simulink model "teleop2_arrows_32"  (Simulink 10.3)
settings: Solver=ode1  StartTime=0.0  StopTime=inf  FixedStep=0.01  RelTol=1e-3  EnableMultiTasking=on
undefined symbols (not defined in the file): gcbh, HIL, Host, JPEG, qc_get_step_size, Video3D, video_display_show
libraries: quarc_library x18
settings Model: Creator=drmadill  LastModifiedBy=Rohan  SimulationMode=external  ExtModeTrigDuration=2
settings SolverCC: PositivePriorityOrder=on
settings DataIOCC: LimitDataPoints=on
settings OptimizationCC: LifeSpan=auto
settings DebuggingCC: SolverPrmCheckMsg=warning
settings HardwareCC: ProdLargestAtomicInteger=Long  ProdLargestAtomicFloat=Double  ProdIntDivRoundTo=Zero  ProdEndianess=LittleEndian  ProdHWDeviceType=ARM Compatible->ARM Cortex
settings RTWCC: Description=QUARC Linux Raspberry Pi 3 Target (QBot 2e) Using Toolchain  SystemTargetFile=quarc_linux_pi_3.tlc  TemplateMakefile=quarc_default_tmf  Toolchain=QUARC linux_pi_3 | gmake (64-bit Windows)  BuildConfiguration=Faster Runs
settings STFCustomTargetCC: ConcurrentExecutionCompliant=on  UseToolchainInfoCompliant=on  SystemTargetFile=quarc_linux_pi_3.tlc
settings GRTTargetCC: ParMdlRefBuildCompliant=off  CompOptLevelCompliant=off  MatFileLogging=off  CPPClassGenCompliant=off  ExtMode=on  ExtModeMexFile=quarc_comm  ExtModeMexArgs='-w -d /tmp -uri %u', 'tcpip://192.168.2.32:17001'
settings ConfigComp: CovSFcnEnable=off

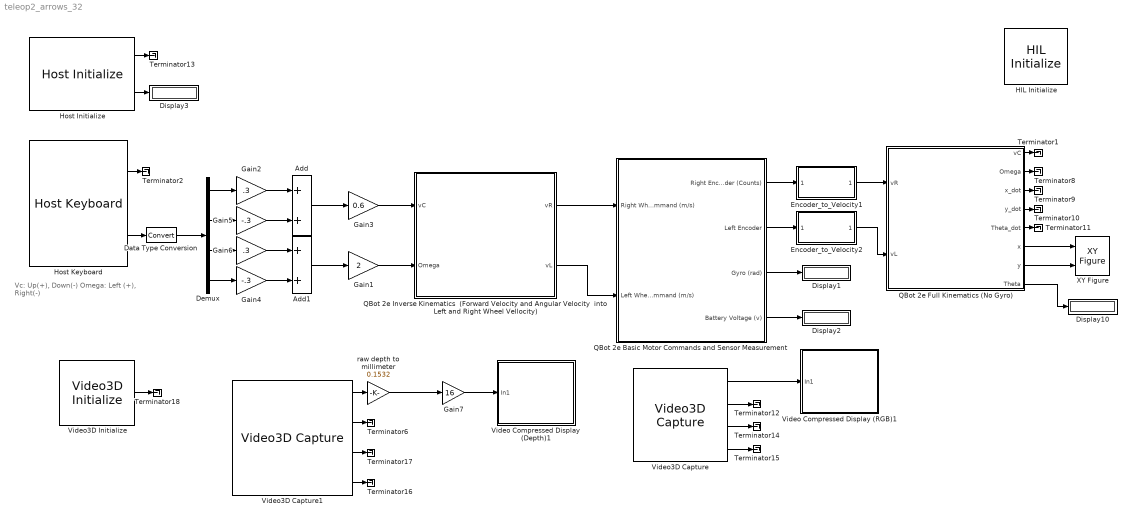
== system teleop2_arrows_32 ==
  note: Vc: Up(+), Down(-)
      | Omega: Left (+), Right(-)
  Add : Sum
  Add1 : Sum
  Data Type Conversion : DataTypeConversion
  Demux : Demux
  Display{1..3,10} (4 alike) : Display
  Encoder_to_Velocity1 : Subsystem
  Encoder_to_Velocity2 : Subsystem
  Gain1 : Gain  Gain=2
  Gain2 : Gain  Gain=.3
  Gain3 : Gain  Gain=0.6
  Gain4 : Gain  Gain=-.3
  Gain5 : Gain  Gain=-.3
  Gain6 : Gain  Gain=.3
  Gain7 : Gain  Gain=16  OutDataTypeStr=uint16
  HIL Initialize : quarc_library/Data Acquisition/Generic/Configuration/HIL Initialize  Priority=-99  object_name=HIL-1  board_type=qbot2e  board_number=0  board_options=pwm0_en=1;pwm0_pin=12;pwm1_en=1;pwm1_pin=13;  exclusive=off  active=off  hardware_clocks=[]  clock_modes=[]  initial_clock_frequencies=[]  set_clock_params_at_start=off  set_clock_params_at_switch_in=off  set_clock_frequencies_at_start=off  set_clock_frequencies_at_switch_in=off  analog_input_channels=[0:5]  analog_input_configurations=[]  analog_input_maximums=[16.5 3.3 3.3 3.3 3.3 3.3]  analog_input_minimums=[0 0 0 0 0 0]  set_analog_input_params_at_start=off  set_analog_input_params_at_switch_in=off  analog_output_channels=[]  analog_output_maximums=[]  analog_output_minimums=[]  initial_analog_outputs=[]  final_analog_outputs=[]  watchdog_analog_outputs=[]  set_analog_output_params_at_start=off  set_analog_output_params_at_switch_in=off  set_analog_outputs_at_start=off  set_analog_outputs_at_switch_in=off  set_analog_outputs_at_terminate=off  set_analog_outputs_at_switch_out=off  set_analog_outputs_on_watchdog=off  digital_input_channels=[28:58]  digital_output_channels=[28:31]  digital_output_configuration=[]  initial_digital_outputs=[0]  final_digital_outputs=[0]  watchdog_digital_outputs=[]  set_digital_output_params_at_start=off  set_digital_output_params_at_switch_in=off  set_digital_outputs_at_start=on  set_digital_outputs_at_switch_in=off  set_digital_outputs_at_terminate=on  set_digital_outputs_at_switch_out=off  set_digital_outputs_on_watchdog=off  encoder_channels=[0:1]  quadrature=[4]  encoder_filter_frequency=[]  initial_encoder_counts=[0]  set_encoder_params_at_start=on  set_encoder_params_at_switch_in=off  set_encoder_counts_at_start=on  set_encoder_counts_at_switch_in=off  pwm_channels=[0:1]  pwm_modes=0  pwm_frequency=100e6 / 4095  pwm_configuration=[0]  pwm_alignment=[0]  pwm_polarity=[1]  pwm_leading_deadband=[]  pwm_trailing_deadband=[]  initial_pwm_outputs=[0]  final_pwm_outputs=[0]  watchdog_pwm_outputs=[]  set_pwm_params_at_start=on  set_pwm_params_at_switch_in=off  set_pwm_outputs_at_start=on  set_pwm_outputs_at_switch_in=off  set_pwm_outputs_at_terminate=on  set_pwm_outputs_at_switch_out=off  set_pwm_outputs_on_watchdog=off  other_output_channels=[2000:2001 14000 16000]  initial_other_outputs=[0 0 0 7]  final_other_outputs=[0 0 0 7]  watchdog_other_outputs=[]  set_other_outputs_at_start=on  set_other_outputs_at_switch_in=off  set_other_outputs_at_terminate=on  set_other_outputs_at_switch_out=off  set_other_outputs_on_watchdog=off
  Host Initialize : quarc_library/Devices/Peripherals/Host/Host Initialize  object_name=Host-1  uri_source=Use external mode communications  uri=tcpip://192.168.2.104:17001  apply_uri_to_all_configs=on  send_buffer_size=1000  receive_buffer_size=1000  thread_priority=0  run_client=on  use_window=off  window_position=[]  sample_time=qc_get_step_size  active=on
      settings: SourceProductName=QUARC Targets
  Host Keyboard : quarc_library/Devices/Peripherals/Host/Host Keyboard  object_name=Host-1  virtual_key="[38  40  37  39]"  sample_time=qc_get_step_size  enabled=on  debug_mode=off
      settings: SourceProductName=QUARC Targets
  QBot 2e Basic Motor Commands and Sensor Measurement : Subsystem
  QBot 2e Full Kinematics (No Gyro) : Subsystem
  QBot 2e Inverse Kinematics  (Forward Velocity and Angular Velocity  into Left and Right Wheel Vellocity) : Subsystem
  Terminator{1..2,6,8..18} (14 alike) : Terminator
  Video Compressed Display (Depth)1 : Subsystem  LoadFcn=set_param(gcbh, 'UserData', gcb);  StartFcn=video_display_show([gcb, '/Video Display'], 'add', gcb);  mask(Video Compressed Display){algorithm=JPEG, quality=50, sample_time=-1, use_hardware=on}
      mask prompts: algorithm "Compression algorithm:"; quality "Compression quality (0-100):"; sample_time "Sample time (seconds):"; use_hardware "Use hardware acceleration for video display"
      mask help: Displays a video stream on the host, using compression to minimize bandwidth.
      mask init:
      | qc_set_display('Video\nCompressed\nDisplay');
      settings: UndoDeleteFcn=set_param(gcbh, 'UserData', gcb);  OpenFcn=video_display_show([gcb, '/Video Display'], 'show', gcb);  PreDeleteFcn=video_display_show([gcb, '/Video Display'], 'delete');
      settings: CopyFcn=|
      | set_param(gcbh, 'UserData', gcb);
      | set_param(gcbh, 'LinkStatus', 'none');
      settings: NameChangeFcn=|
      | video_display_show([get_param(gcbh, 'UserData'), '/Video Display'], 'rename', [gcb, '/Video Display']);
      | video_display_show([gcb, '/Video Display'], 'add', gcb);
      | set_param(gcbh, 'UserData', gcb);
      mask Help: web(qc_get_block_help_path(gcb));
      mask TypeOptions algorithm: Image Compress/algorithm
      mask TypeOptions quality: Image Compress/quality
      mask TypeOptions sample_time: Video Display/sample_time
      mask TypeOptions use_hardware: Video Display/use_hardware
      mask Display:
      | patch([0.98591 0.98591 0.62618 0.59072 0.56147   0.536   0.536  0.5441 0.56912 0.59207 0.60881 0.62276 0.63527 0.64364  0.6485  0.6485 0.64706 0.64499 0.63662 0.62411 0.61232 0.59837 0.58307 0.56147   0.536   0.536  0.5441  0.5747 0.60953 0.63662 0.67001  0.7034 0.72851 0.75425 0.77927 0.80294 0.82454 0.84119 0.85865 0.87395 0.88574 0.89339  0.8969 0.89969 0.89969 0.89267  0.8816 0.87044 0.85649  0.8384 0.81824 0.80294 0.78764 0.77513 0.76676 0.75776 0.76397 0.77513 0.79178 0.80987 0.82796 0.84326 0.86207 0.98528],[0.18689 0.05522 0.05522 0.05171 0.05171    0.05 0.18338 0.18338 0.19148 0.20435 0.22298 0.24863 0.28589 0.33125 0.38138 0.55139 0.59801 0.63761 0.68189 0.72149 0.74939 0.76694 0.77855 0.79367 0.79952 0.92768 0.92768 0.92768 0.92417 0.92066 0.91364  0.9032 0.89384 0.88106 0.86594 0.85073 0.82634 0.80537 0.77855 0.74363 0.70403 0.65858 0.61079 0.59099 0.41513 0.37202 0.31847 0.29048 0.25556 0.23342  0.2102 0.19382 0.18221 0.17285 0.16943 0.16124  0.1589 0.16241 0.16709 0.17168  0.1787 0.18221 0.18689 0.18689],[0.9,0.90,0.91])
      | patch([0.536 0.52601 0.46823 0.44528 0.41603 0.39101 0.35555 0.33116 0.31451 0.29291  0.2804 0.26717 0.25322 0.23999 0.22406 0.20732 0.19337 0.17528 0.15935 0.14396 0.13217 0.11759 0.10922 0.10085 0.09671 0.09392 0.09041 0.08906 0.08906 0.09464  0.0995 0.10778 0.11894 0.13145 0.14675 0.16349 0.17672 0.19409 0.20732 0.22406 0.23999 0.26159 0.27833 0.29849 0.31793 0.33602 0.35411 0.37085 0.39245 0.41603   0.536   0.536 0.53159 0.46409   0.446 0.42026 0.39587 0.37571 0.36113 0.34925 0.34088 0.33809 0.33809 0.34088 0.34583 0.35627 0.36392 0.38129 0.39587 0.41117 0.42719 0.44672  0.4676 0.48353 0.48353 0.52394   0.536],[0.05 0.04829 0.04712 0.04712 0.04829 0.05063 0.05405 0.05873 0.06107 0.06692 0.07043 0.07619 0.08087 0.08672 0.09482 0.10652 0.11696 0.13325  0.1508 0.17168 0.19499 0.22415 0.25439 0.28472 0.31379 0.35456 0.38489 0.41513 0.58055 0.63878 0.68774 0.72149 0.75641 0.78089 0.80537 0.82859 0.84029 0.85658 0.86594 0.87404  0.8834 0.89267 0.90086 0.90788 0.91247 0.91832 0.92066   0.923 0.92651 0.92768 0.92768 0.79952 0.79952 0.79952 0.79718 0.78899 0.77153 0.75056 0.72149 0.68072 0.62249  0.5549 0.41396 0.37085 0.33242 0.28121 0.25205 0.22181 0.20552 0.19499 0.18572 0.18221 0.17753 0.17636 0.17753  0.1787  0.1787],[0.9,0.90,0.91])
      | disp('Video\nCompressed\nDisplay');
  Video Compressed Display (RGB)1 : Subsystem  LoadFcn=set_param(gcbh, 'UserData', gcb);  StartFcn=video_display_show([gcb, '/Video Display'], 'add', gcb);  mask(Video Compressed Display){algorithm=JPEG, quality=50, sample_time=-1, use_hardware=on}
      mask prompts: algorithm "Compression algorithm:"; quality "Compression quality (0-100):"; sample_time "Sample time (seconds):"; use_hardware "Use hardware acceleration for video display"
      mask help: Displays a video stream on the host, using compression to minimize bandwidth.
      mask init:
      | qc_set_display('Video\nCompressed\nDisplay');
      settings: UndoDeleteFcn=set_param(gcbh, 'UserData', gcb);  OpenFcn=video_display_show([gcb, '/Video Display'], 'show', gcb);  PreDeleteFcn=video_display_show([gcb, '/Video Display'], 'delete');
      settings: CopyFcn=|
      | set_param(gcbh, 'UserData', gcb);
      | set_param(gcbh, 'LinkStatus', 'none');
      settings: NameChangeFcn=|
      | video_display_show([get_param(gcbh, 'UserData'), '/Video Display'], 'rename', [gcb, '/Video Display']);
      | video_display_show([gcb, '/Video Display'], 'add', gcb);
      | set_param(gcbh, 'UserData', gcb);
      mask Help: web(qc_get_block_help_path(gcb));
      mask TypeOptions algorithm: Image Compress/algorithm
      mask TypeOptions quality: Image Compress/quality
      mask TypeOptions sample_time: Video Display/sample_time
      mask TypeOptions use_hardware: Video Display/use_hardware
      mask Display:
      | patch([0.98591 0.98591 0.62618 0.59072 0.56147   0.536   0.536  0.5441 0.56912 0.59207 0.60881 0.62276 0.63527 0.64364  0.6485  0.6485 0.64706 0.64499 0.63662 0.62411 0.61232 0.59837 0.58307 0.56147   0.536   0.536  0.5441  0.5747 0.60953 0.63662 0.67001  0.7034 0.72851 0.75425 0.77927 0.80294 0.82454 0.84119 0.85865 0.87395 0.88574 0.89339  0.8969 0.89969 0.89969 0.89267  0.8816 0.87044 0.85649  0.8384 0.81824 0.80294 0.78764 0.77513 0.76676 0.75776 0.76397 0.77513 0.79178 0.80987 0.82796 0.84326 0.86207 0.98528],[0.18689 0.05522 0.05522 0.05171 0.05171    0.05 0.18338 0.18338 0.19148 0.20435 0.22298 0.24863 0.28589 0.33125 0.38138 0.55139 0.59801 0.63761 0.68189 0.72149 0.74939 0.76694 0.77855 0.79367 0.79952 0.92768 0.92768 0.92768 0.92417 0.92066 0.91364  0.9032 0.89384 0.88106 0.86594 0.85073 0.82634 0.80537 0.77855 0.74363 0.70403 0.65858 0.61079 0.59099 0.41513 0.37202 0.31847 0.29048 0.25556 0.23342  0.2102 0.19382 0.18221 0.17285 0.16943 0.16124  0.1589 0.16241 0.16709 0.17168  0.1787 0.18221 0.18689 0.18689],[0.9,0.90,0.91])
      | patch([0.536 0.52601 0.46823 0.44528 0.41603 0.39101 0.35555 0.33116 0.31451 0.29291  0.2804 0.26717 0.25322 0.23999 0.22406 0.20732 0.19337 0.17528 0.15935 0.14396 0.13217 0.11759 0.10922 0.10085 0.09671 0.09392 0.09041 0.08906 0.08906 0.09464  0.0995 0.10778 0.11894 0.13145 0.14675 0.16349 0.17672 0.19409 0.20732 0.22406 0.23999 0.26159 0.27833 0.29849 0.31793 0.33602 0.35411 0.37085 0.39245 0.41603   0.536   0.536 0.53159 0.46409   0.446 0.42026 0.39587 0.37571 0.36113 0.34925 0.34088 0.33809 0.33809 0.34088 0.34583 0.35627 0.36392 0.38129 0.39587 0.41117 0.42719 0.44672  0.4676 0.48353 0.48353 0.52394   0.536],[0.05 0.04829 0.04712 0.04712 0.04829 0.05063 0.05405 0.05873 0.06107 0.06692 0.07043 0.07619 0.08087 0.08672 0.09482 0.10652 0.11696 0.13325  0.1508 0.17168 0.19499 0.22415 0.25439 0.28472 0.31379 0.35456 0.38489 0.41513 0.58055 0.63878 0.68774 0.72149 0.75641 0.78089 0.80537 0.82859 0.84029 0.85658 0.86594 0.87404  0.8834 0.89267 0.90086 0.90788 0.91247 0.91832 0.92066   0.923 0.92651 0.92768 0.92768 0.79952 0.79952 0.79952 0.79718 0.78899 0.77153 0.75056 0.72149 0.68072 0.62249  0.5549 0.41396 0.37085 0.33242 0.28121 0.25205 0.22181 0.20552 0.19499 0.18572 0.18221 0.17753 0.17636 0.17753  0.1787  0.1787],[0.9,0.90,0.91])
      | disp('Video\nCompressed\nDisplay');
  Video3D Capture : quarc_library/Multimedia/Video3D Capture  object_name=Video3D-1  stream_type=RGB  stream_index=0  resolution=640 x 480  width=640  height=480  output_format=MATLAB RGB (HxWx3)  data_type=uint8  sample_time=qc_get_step_size * ceil(0.033 / qc_get_step_size)  brightness_override=off  brightness=50.0  contrast_override=off  contrast=50.0  hue_override=off  hue=50.0  saturation_override=off  saturation=50.0  sharpness_override=off  sharpness=50.0  gamma_override=off  gamma=50.0  gain_override=off  gain=50.0  backlightcompensation_override=off  backlightcompensation=50.0  whitebalance_override=Automatic white balance  whitebalance=50.0  exposure_override=Automatic exposure  exposure=30.0  emitter=Enable laser emitter  preset=Do not set camera presets
  Video3D Capture1 : quarc_library/Multimedia/Video3D Capture  object_name=Video3D-1  stream_type=Depth  stream_index=0  resolution=640 x 480  width=640  height=480  output_format=MATLAB greyscale (HxW)  data_type=uint16  sample_time=qc_get_step_size * ceil(0.033 / qc_get_step_size)  brightness_override=off  brightness=50.0  contrast_override=off  contrast=50.0  hue_override=off  hue=50.0  saturation_override=off  saturation=50.0  sharpness_override=off  sharpness=50.0  gamma_override=off  gamma=50.0  gain_override=off  gain=50.0  backlightcompensation_override=off  backlightcompensation=50.0  whitebalance_override=Automatic white balance  whitebalance=50.0  exposure_override=Automatic exposure  exposure=30.0  emitter=Enable laser emitter  preset=Do not set camera presets
  Video3D Initialize : quarc_library/Multimedia/Video3D Initialize  object_name=Video3D-1  source=Device  identifier=0  file=sample.bag  sample_time=qc_get_step_size * ceil(0.033 / qc_get_step_size)  active=on
  XY Figure : quarc_library/Sinks/Figures/XY Figure  figure_mode=Use figure window  figure_tag=figure1  axes_tag=axes1  plot_mode=Time-based  minimum_x=-1  maximum_x=1  minimum_y=-1  maximum_y=1  buffer_size=1000  update_rate=100  initial_position="581  184  710  615"  initial_visibility=off  sample_time=-1
      settings: SourceProductName=QUARC Targets
  raw depth to millimeter : Gain  Gain=0.1532
  wires:
  Host Initialize/2 -> Display3/1
  Host Initialize/1 -> Terminator13/1
  QBot 2e Basic Motor Commands and Sensor Measurement/2(Left Encoder) -> Encoder_to_Velocity2/1(Encoder)
  QBot 2e Full Kinematics (No Gyro)/8(Theta) -> Display10/1
  QBot 2e Full Kinematics (No Gyro)/7(y) -> XY Figure/2
  QBot 2e Full Kinematics (No Gyro)/6(x) -> XY Figure/1
  Encoder_to_Velocity1/1(Velocity) -> QBot 2e Full Kinematics (No Gyro)/1(vR)
  Encoder_to_Velocity2/1(Velocity) -> QBot 2e Full Kinematics (No Gyro)/2(vL)
  QBot 2e Inverse Kinematics  (Forward Velocity and Angular Velocity  into Left and Right Wheel Vellocity)/1(vR) -> QBot 2e Basic Motor Commands and Sensor Measurement/1(Right Wheel Command (m/s))
  Gain3/1 -> QBot 2e Inverse Kinematics  (Forward Velocity and Angular Velocity  into Left and Right Wheel Vellocity)/1(vC)
  QBot 2e Full Kinematics (No Gyro)/2(Omega) -> Terminator8/1
  QBot 2e Full Kinematics (No Gyro)/3(x_dot) -> Terminator9/1
  QBot 2e Full Kinematics (No Gyro)/4(y_dot) -> Terminator10/1
  QBot 2e Full Kinematics (No Gyro)/5(Theta_dot) -> Terminator11/1
  Host Keyboard/2 -> Data Type Conversion/1
  Demux/1 -> Gain2/1
  Demux/4 -> Gain4/1
  Gain2/1 -> Add/1
  Add/1 -> Gain3/1
  Demux/2 -> Gain5/1
  Demux/3 -> Gain6/1
  Add1/1 -> Gain1/1
  Data Type Conversion/1 -> Demux/1
  Gain5/1 -> Add/2
  Gain6/1 -> Add1/1
  Gain4/1 -> Add1/2
  QBot 2e Full Kinematics (No Gyro)/1(vC) -> Terminator1/1
  Host Keyboard/1 -> Terminator2/1
  Gain1/1 -> QBot 2e Inverse Kinematics  (Forward Velocity and Angular Velocity  into Left and Right Wheel Vellocity)/2(Omega)
  QBot 2e Inverse Kinematics  (Forward Velocity and Angular Velocity  into Left and Right Wheel Vellocity)/2(vL) -> QBot 2e Basic Motor Commands and Sensor Measurement/2(Left Wheel Command (m/s))
  QBot 2e Basic Motor Commands and Sensor Measurement/1(Right Encoder (Counts)) -> Encoder_to_Velocity1/1(Encoder)
  QBot 2e Basic Motor Commands and Sensor Measurement/3(Gyro (rad)) -> Display1/1
  QBot 2e Basic Motor Commands and Sensor Measurement/4(Battery Voltage (v)) -> Display2/1
  Video3D Capture1/4 -> Terminator16/1
  raw depth to millimeter/1 -> Gain7/1
  Video3D Capture/1 -> Video Compressed Display (RGB)1/1(In1)
  Video3D Capture1/3 -> Terminator17/1
  Video3D Capture/3 -> Terminator14/1
  Gain7/1 -> Video Compressed Display (Depth)1/1(In1)
  Video3D Capture1/1 -> raw depth to millimeter/1
  Video3D Capture/2 -> Terminator12/1
  Video3D Capture1/2 -> Terminator6/1
  Video3D Capture/4 -> Terminator15/1
  Video3D Initialize/1 -> Terminator18/1

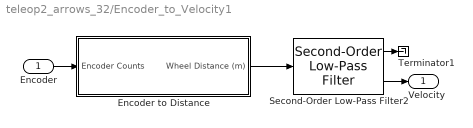
== system teleop2_arrows_32/Encoder_to_Velocity1 ==
  Encoder : Inport
  Encoder to Distance : Subsystem
  Second-Order Low-Pass Filter2 : quarc_library/Continuous/Second-Order Low-Pass Filter  params_source=Internal (dialog parameters)  input_width=10  input_zeta=1  input_init=0
  Terminator1 : Terminator
  Velocity : Outport
  wires:
  Second-Order Low-Pass Filter2/2 -> Velocity/1
  Encoder/1 -> Encoder to Distance/1(Encoder Counts)
  Encoder to Distance/1(Wheel Distance (m)) -> Second-Order Low-Pass Filter2/1
  Second-Order Low-Pass Filter2/1 -> Terminator1/1

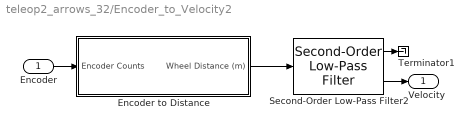
== system teleop2_arrows_32/Encoder_to_Velocity2 ==
  Encoder : Inport
  Encoder to Distance : Subsystem
  Second-Order Low-Pass Filter2 : quarc_library/Continuous/Second-Order Low-Pass Filter  params_source=Internal (dialog parameters)  input_width=10  input_zeta=1  input_init=0
  Terminator1 : Terminator
  Velocity : Outport
  wires:
  Second-Order Low-Pass Filter2/1 -> Terminator1/1
  Encoder to Distance/1(Wheel Distance (m)) -> Second-Order Low-Pass Filter2/1
  Encoder/1 -> Encoder to Distance/1(Encoder Counts)
  Second-Order Low-Pass Filter2/2 -> Velocity/1

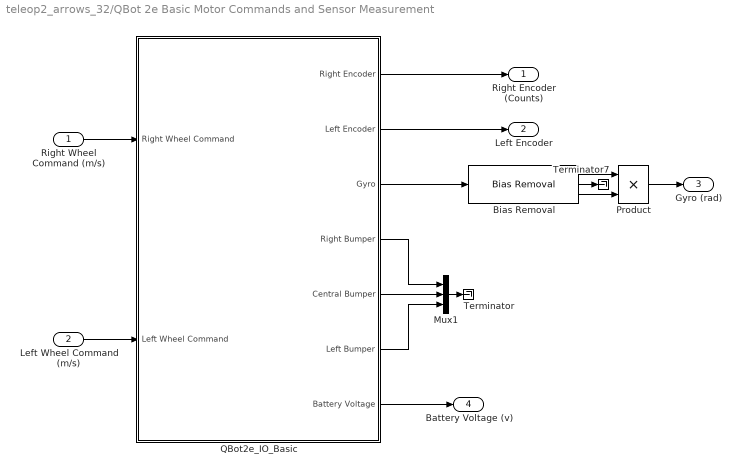
== system teleop2_arrows_32/QBot 2e Basic Motor Commands and Sensor Measurement ==
  Right Wheel Command (m/s) : Inport
  Left Wheel Command (m/s) : Inport  Port=2
  Bias Removal : quarc_library/Discrete/Bias Removal  start_time=3  end_time=4  switch_id=0  sample_time=qc_get_step_size
      settings: SourceProductName=QUARC Targets
  Mux1 : Mux  Inputs=3
  Product : Product  RndMeth=Zero
  QBot2e_IO_Basic : Subsystem
  Terminator : Terminator
  Terminator7 : Terminator
  Right Encoder (Counts) : Outport
  Left Encoder : Outport  Port=2
  Gyro (rad) : Outport  Port=3
  Battery Voltage (v) : Outport  Port=4
  wires:
  QBot2e_IO_Basic/4(Right Bumper) -> Mux1/1
  QBot2e_IO_Basic/5(Central Bumper) -> Mux1/2
  QBot2e_IO_Basic/6(Left Bumper) -> Mux1/3
  Right Wheel Command (m/s)/1 -> QBot2e_IO_Basic/1(Right Wheel Command)
  Left Wheel Command (m/s)/1 -> QBot2e_IO_Basic/2(Left Wheel Command)
  QBot2e_IO_Basic/1(Right Encoder) -> Right Encoder (Counts)/1
  QBot2e_IO_Basic/2(Left Encoder) -> Left Encoder/1
  QBot2e_IO_Basic/7(Battery Voltage) -> Battery Voltage (v)/1
  Bias Removal/2 -> Terminator7/1
  Bias Removal/1 -> Product/1
  Bias Removal/3 -> Product/2
  Product/1 -> Gyro (rad)/1
  QBot2e_IO_Basic/3(Gyro) -> Bias Removal/1
  Mux1/1 -> Terminator/1

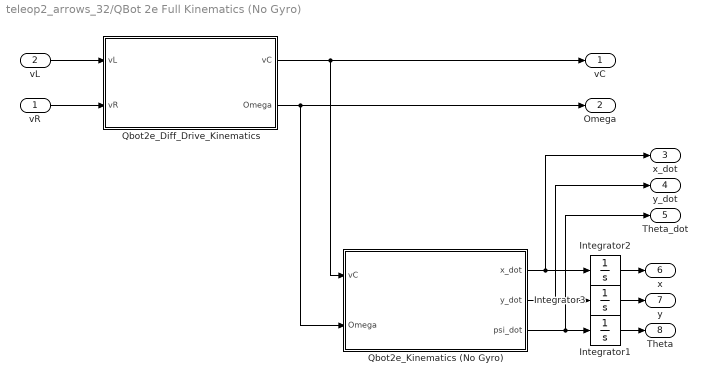
== system teleop2_arrows_32/QBot 2e Full Kinematics (No Gyro) ==
  vR : Inport
  vL : Inport  Port=2
  Integrator1 : Integrator
  Integrator2 : Integrator
  Integrator3 : Integrator
  Qbot2e_Diff_Drive_Kinematics : Subsystem
  Qbot2e_Kinematics (No Gyro) : Subsystem
  vC : Outport
  Omega : Outport  Port=2
  x_dot : Outport  Port=3
  y_dot : Outport  Port=4
  Theta_dot : Outport  Port=5
  x : Outport  Port=6
  y : Outport  Port=7
  Theta : Outport  Port=8
  wires:
  Qbot2e_Diff_Drive_Kinematics/2(Omega) -> Omega/1, Qbot2e_Kinematics (No Gyro)/2(Omega)
  Integrator3/1 -> y/1
  Integrator2/1 -> x/1
  vR/1 -> Qbot2e_Diff_Drive_Kinematics/2(vR)
  vL/1 -> Qbot2e_Diff_Drive_Kinematics/1(vL)
  Qbot2e_Diff_Drive_Kinematics/1(vC) -> vC/1, Qbot2e_Kinematics (No Gyro)/1(vC)
  Qbot2e_Kinematics (No Gyro)/2(y_dot) -> Integrator3/1, y_dot/1
  Qbot2e_Kinematics (No Gyro)/1(x_dot) -> Integrator2/1, x_dot/1
  Qbot2e_Kinematics (No Gyro)/3(psi_dot) -> Integrator1/1, Theta_dot/1
  Integrator1/1 -> Theta/1

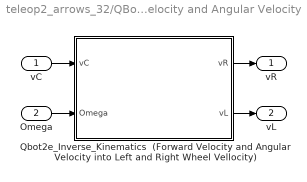
== system teleop2_arrows_32/QBot 2e Inverse Kinematics  (Forward Velocity and Angular Velocity  into Left and Right Wheel Vellocity) ==
  vC : Inport
  Omega : Inport  Port=2
  Qbot2e_Inverse_Kinematics  (Forward Velocity and Angular Velocity into Left and Right Wheel Vellocity) : MATLAB Function  TreatAsAtomicUnit=on
  vR : Outport
  vL : Outport  Port=2
  wires:
  vC/1 -> Qbot2e_Inverse_Kinematics  (Forward Velocity and Angular Velocity into Left and Right Wheel Vellocity)/1(vC)
  Qbot2e_Inverse_Kinematics  (Forward Velocity and Angular Velocity into Left and Right Wheel Vellocity)/1(vR) -> vR/1
  Omega/1 -> Qbot2e_Inverse_Kinematics  (Forward Velocity and Angular Velocity into Left and Right Wheel Vellocity)/2(Omega)
  Qbot2e_Inverse_Kinematics  (Forward Velocity and Angular Velocity into Left and Right Wheel Vellocity)/2(vL) -> vL/1

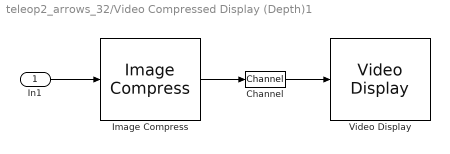
== system teleop2_arrows_32/Video Compressed Display (Depth)1 ==
  In1 : Inport
  Channel : quarc_library/Signal Routing/Channel  channel=0  buffer_size=1
  Image Compress : quarc_library/Image Processing/Generic/Image Compress  algorithm=JPEG  source=Internal dialog parameter  quality=quality  output_dim=-1
  Video Display : quarc_library/Multimedia/Video Display  Tag=|  sample_time=sample_time  use_hardware=on
      | teleop2_arrows_32/Video Compressed
      | Display (Depth)1/Video Display
  wires:
  Image Compress/1 -> Channel/1
  In1/1 -> Image Compress/1
  Channel/1 -> Video Display/1

== system teleop2_arrows_32/Video Compressed Display (RGB)1 ==
  In1 : Inport
  Channel : quarc_library/Signal Routing/Channel  channel=1  buffer_size=1
  Image Compress : quarc_library/Image Processing/Generic/Image Compress  algorithm=JPEG  source=Internal dialog parameter  quality=quality  output_dim=-1
  Video Display : quarc_library/Multimedia/Video Display  Tag=|  sample_time=sample_time  use_hardware=on
      | teleop2_arrows_32/Video Compressed
      | Display (RGB)1/Video Display
  wires:
  Channel/1 -> Video Display/1
  In1/1 -> Image Compress/1
  Image Compress/1 -> Channel/1

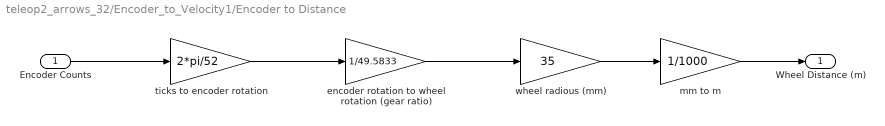
== system teleop2_arrows_32/Encoder_to_Velocity1/Encoder to Distance ==
  Encoder Counts : Inport
  " encoder rotation to wheel rotation (gear ratio)" : Gain  Gain=1/49.5833
  mm to m : Gain  Gain=1/1000
  ticks to encoder rotation : Gain  Gain=2*pi/52
  wheel radious (mm) : Gain  Gain=35
  Wheel Distance (m) : Outport
  wires:
  mm to m/1 -> Wheel Distance (m)/1
  wheel radious (mm)/1 -> mm to m/1
  " encoder rotation to wheel rotation (gear ratio)"/1 -> wheel radious (mm)/1
  ticks to encoder rotation/1 -> " encoder rotation to wheel rotation (gear ratio)"/1
  Encoder Counts/1 -> ticks to encoder rotation/1

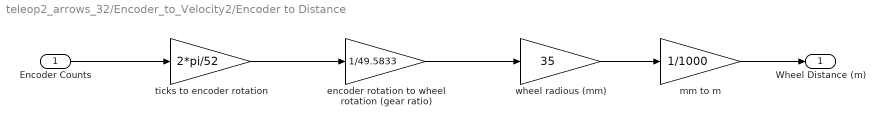
== system teleop2_arrows_32/Encoder_to_Velocity2/Encoder to Distance ==
  Encoder Counts : Inport
  " encoder rotation to wheel rotation (gear ratio)" : Gain  Gain=1/49.5833
  mm to m : Gain  Gain=1/1000
  ticks to encoder rotation : Gain  Gain=2*pi/52
  wheel radious (mm) : Gain  Gain=35
  Wheel Distance (m) : Outport
  wires:
  Encoder Counts/1 -> ticks to encoder rotation/1
  ticks to encoder rotation/1 -> " encoder rotation to wheel rotation (gear ratio)"/1
  " encoder rotation to wheel rotation (gear ratio)"/1 -> wheel radious (mm)/1
  wheel radious (mm)/1 -> mm to m/1
  mm to m/1 -> Wheel Distance (m)/1

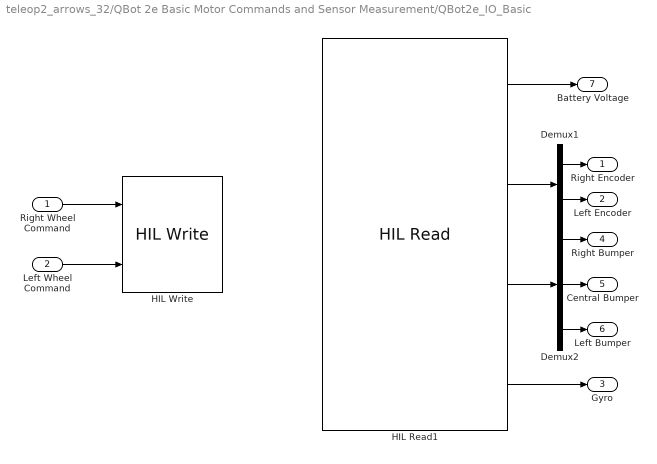
== system teleop2_arrows_32/QBot 2e Basic Motor Commands and Sensor Measurement/QBot2e_IO_Basic ==
  Right Wheel Command : Inport
  Left Wheel Command : Inport  Port=2
  Demux1 : Demux  Outputs=2
  Demux2 : Demux  Outputs=3
  HIL Read1 : quarc_library/Data Acquisition/Generic/Immediate I//O/HIL Read  object_name=HIL-1  analog_channels=[0]  encoder_channels=[0:1]  digital_channels=[28:30]  other_channels=[1002]  sample_time=qc_get_step_size  active=on  vector_output=on  data_type_mode=Inherit via back propagation  encoder_data_type=double  digital_data_type=boolean
  HIL Write : quarc_library/Data Acquisition/Generic/Immediate I//O/HIL Write  object_name=HIL-1  analog_channels=[]  pwm_channels=[]  digital_channels=[]  other_channels=[2000:2001]  sample_time=-1  active=on  vector_input=off
  Right Encoder : Outport
  Left Encoder : Outport  Port=2
  Gyro : Outport  Port=3
  Right Bumper : Outport  Port=4
  Central Bumper : Outport  Port=5
  Left Bumper : Outport  Port=6
  Battery Voltage : Outport  Port=7
  wires:
  HIL Read1/1 -> Battery Voltage/1
  HIL Read1/3 -> Demux2/1
  HIL Read1/4 -> Gyro/1
  Demux1/1 -> Right Encoder/1
  Demux1/2 -> Left Encoder/1
  Right Wheel Command/1 -> HIL Write/1
  Left Wheel Command/1 -> HIL Write/2
  HIL Read1/2 -> Demux1/1
  Demux2/1 -> Right Bumper/1
  Demux2/2 -> Central Bumper/1
  Demux2/3 -> Left Bumper/1

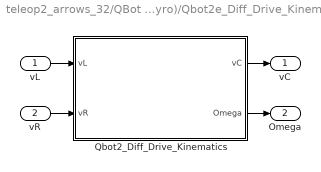
== system teleop2_arrows_32/QBot 2e Full Kinematics (No Gyro)/Qbot2e_Diff_Drive_Kinematics ==
  vL : Inport
  vR : Inport  Port=2
  Qbot2_Diff_Drive_Kinematics : MATLAB Function  TreatAsAtomicUnit=on
  vC : Outport
  Omega : Outport  Port=2
  wires:
  Qbot2_Diff_Drive_Kinematics/2(Omega) -> Omega/1
  vR/1 -> Qbot2_Diff_Drive_Kinematics/2(vR)
  Qbot2_Diff_Drive_Kinematics/1(vC) -> vC/1
  vL/1 -> Qbot2_Diff_Drive_Kinematics/1(vL)

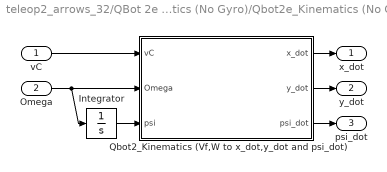
== system teleop2_arrows_32/QBot 2e Full Kinematics (No Gyro)/Qbot2e_Kinematics (No Gyro) ==
  vC : Inport
  Omega : Inport  Port=2
  Integrator : Integrator
  Qbot2_Kinematics (Vf,W to x_dot,y_dot and psi_dot) : MATLAB Function  TreatAsAtomicUnit=on
  x_dot : Outport
  y_dot : Outport  Port=2
  psi_dot : Outport  Port=3
  wires:
  Qbot2_Kinematics (Vf,W to x_dot,y_dot and psi_dot)/2(y_dot) -> y_dot/1
  Omega/1 -> Qbot2_Kinematics (Vf,W to x_dot,y_dot and psi_dot)/2(Omega), Integrator/1
  Qbot2_Kinematics (Vf,W to x_dot,y_dot and psi_dot)/1(x_dot) -> x_dot/1
  vC/1 -> Qbot2_Kinematics (Vf,W to x_dot,y_dot and psi_dot)/1(vC)
  Integrator/1 -> Qbot2_Kinematics (Vf,W to x_dot,y_dot and psi_dot)/3(psi)
  Qbot2_Kinematics (Vf,W to x_dot,y_dot and psi_dot)/3(psi_dot) -> psi_dot/1

== matlab function QBot 2e Full Kinematics (No Gyro)/Qbot2e_Diff_Drive_Kinematics/Qbot2_Diff_Drive_Kinematics ==
  data: vL input double; vC output double; vR input double; Omega output double
function [vC,Omega] = fcn(vL,vR)
%#codegen

d= 0.235;

vC=0.5*(vL+vR);
Omega=(1/d)*(vR-vL);

== matlab function QBot 2e Full Kinematics (No Gyro)/Qbot2e_Kinematics (No Gyro)/Qbot2_Kinematics (Vf,W to x_dot,y_dot and psi_dot) ==
  data: vC input double; x_dot output double; Omega input double; y_dot output double; psi input double; psi_dot output double
function [x_dot,y_dot,psi_dot] = fcn(vC,Omega,psi)
%#codegen


x_dot=cos(psi)*vC;
y_dot=sin(psi)*vC;
psi_dot= Omega;

== matlab function QBot 2e Inverse Kinematics (Forward Velocity and Angular Velocity into Left and Right Wheel Vellocity)/Qbot2e_Inverse_Kinematics (Forward Velocity and Angular Velocity into Left and Right Wheel Vellocity) ==
  data: vR output double; vL output double; vC input double; Omega input double
function [vR,vL] = fcn(vC , Omega)
%#codegen

d=0.235; 


vR = vC + Omega*d/2;
vL= vC - Omega*d/2;
